simulink model "zaj_3_rd"  (R2015a)
settings: Solver=ode4  StartTime=0.0  StopTime=600  FixedStep=0.1  RelTol=1e-3
settings Model: Creator=Student  LastModifiedBy=lenovo
settings DataIOCC: InspectSignalLogs=on

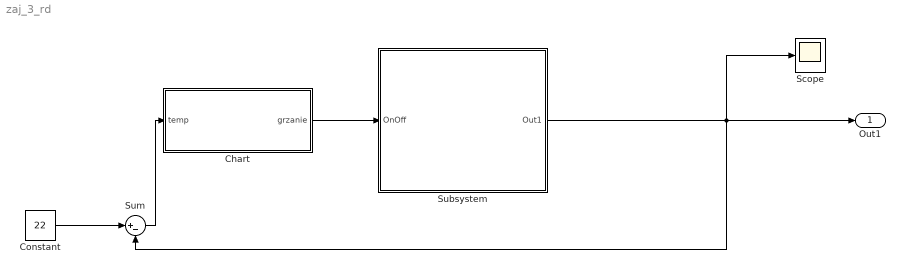
== system zaj_3_rd ==
  Chart : Stateflow chart  TreatAsAtomicUnit=on
  Constant : Constant  Value=22
  Scope : Scope
      settings: TickLabels=on  TimeRange=600  YMax=25  SaveName=ScopeData2
  Subsystem : Subsystem
  Sum : Sum  Inputs=|+-
  Out1 : Outport
  wires:
  Subsystem/1(Out1) -> Sum/2, Out1/1, Scope/1
  Constant/1 -> Sum/1
  Sum/1 -> Chart/1(temp)
  Chart/1(grzanie) -> Subsystem/1(OnOff)

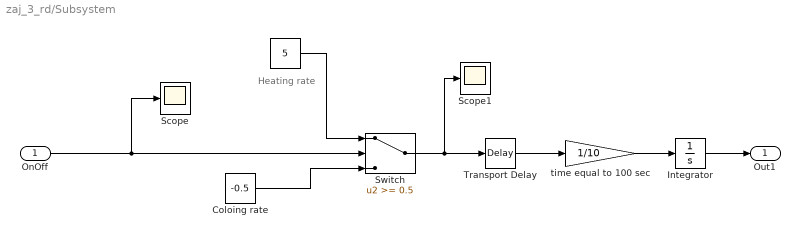
== system zaj_3_rd/Subsystem ==
  note: Heating rate
  OnOff : Inport
  " " : Constant  Value=5
  Coloing rate : Constant  Value=-0.5
  Integrator : Integrator
  Scope : Scope
  Scope1 : Scope
  Switch : Switch  Threshold=0.5
  Transport Delay : TransportDelay
  time equal to 100 sec : Gain  Gain=1/10
  Out1 : Outport
  wires:
  OnOff/1 -> Switch/2, Scope/1
  time equal to 100 sec/1 -> Integrator/1
  Transport Delay/1 -> time equal to 100 sec/1
  Integrator/1 -> Out1/1
  Coloing rate/1 -> Switch/3
  " "/1 -> Switch/1
  Switch/1 -> Scope1/1, Transport Delay/1

== stateflow chart zaj_3_rd/Chart ==
  state On
    during: grzanie=1;
  state Off
    during:grzanie=0;
  On -> Off : [temp<=0]
  Off -> On : [temp>0]
  (default) -> Off
  data: temp input; grzanie output
